simulink model "fuelCycle_Abdou"  (R2022b)
settings: Solver=VariableStepAuto  StartTime=0.0  StopTime=sim_time  RelTol=1e-4
values from neighbouring files (symbols this model uses):
  AF = 90    [BOTH_scenario_inputData.m]    (also in FC_scenario_inputData.m; PO_scenario_inputData.m = 0.7; inputData.m = 70; parametric_analysis_AF.m = AF_array(i))
  eta2 = 0.95    [BOTH_scenario_inputData.m]    (also in FC_scenario_inputData.m; PO_scenario_inputData.m; inputData.m; parametric_analysis_eta_tes.m = eta_tes_array(i))
  f53 = 0.33    [BOTH_scenario_inputData.m]    (also in FC_scenario_inputData.m; PO_scenario_inputData.m; inputData.m; worst_case_InputData.m)
  f54 = 1 - f51 - f53 - f56    (= 0.3399)    [BOTH_scenario_inputData.m]    (also in FC_scenario_inputData.m; PO_scenario_inputData.m; inputData.m; worst_case_InputData.m)
  f56 = 1e-4    (= 0.0001)    [BOTH_scenario_inputData.m]    (also in FC_scenario_inputData.m; PO_scenario_inputData.m; inputData.m; worst_case_InputData.m)
  f96 = 0.1    [BOTH_scenario_inputData.m]    (also in FC_scenario_inputData.m; PO_scenario_inputData.m; inputData.m; worst_case_InputData.m)
  f_dir = 0.7    [BOTH_scenario_inputData.m]    (also in FC_scenario_inputData.m; PO_scenario_inputData.m = 0.3; inputData.m = 0.3; parametric_analysis_f_dir.m = f_dir_array(i))
  fp3 = 1e-4    (= 0.0001)    [BOTH_scenario_inputData.m]    (also in FC_scenario_inputData.m; PO_scenario_inputData.m; inputData.m; parametric_analysis_f_p.m = f_p(i) / 2)
  fp4 = 1e-4    (= 0.0001)    [BOTH_scenario_inputData.m]    (also in FC_scenario_inputData.m; PO_scenario_inputData.m; inputData.m; parametric_analysis_f_p.m = f_p(i) / 2)
  I_s_0 = 1.4    [fuelCycleSimulator.m]    (also in parametric_analysis_AF.m = 0.8; parametric_analysis_epsi.m = 0.8; parametric_analysis_eta_tes.m = 0.8; parametric_analysis_f_dir.m = 0.8)
  lambda = 1.73e-9    (= 1.73e-09)    [BOTH_scenario_inputData.m]    (also in FC_scenario_inputData.m; PO_scenario_inputData.m; inputData.m; worst_case_InputData.m)
  N_dot = 8.99e-7    (= 8.99e-07)    [BOTH_scenario_inputData.m]    (also in FC_scenario_inputData.m = 9.3e-07; PO_scenario_inputData.m = 9.3e-07; inputData.m; worst_case_InputData.m = 9.3e-07)
  T1 = 1/((1 + epsi)/tau1 + lambda)    [BOTH_scenario_inputData.m]    (also in FC_scenario_inputData.m; PO_scenario_inputData.m; inputData.m; parametric_analysis_epsi.m)
  T12 = 1/((1 + epsi)/tau12 + lambda)    [BOTH_scenario_inputData.m]    (also in FC_scenario_inputData.m; PO_scenario_inputData.m; inputData.m; parametric_analysis_epsi.m)
  T2 = 1/((1 + epsi)/tau2 + lambda)    [BOTH_scenario_inputData.m]    (also in FC_scenario_inputData.m; PO_scenario_inputData.m; inputData.m; parametric_analysis_epsi.m)
  T3 = 1/((1 + 0)/tau3 + lambda)    [BOTH_scenario_inputData.m]    (also in FC_scenario_inputData.m; PO_scenario_inputData.m; inputData.m; parametric_analysis_epsi.m)
  T4 = 1/((1 + 0)/tau4 + lambda)    [BOTH_scenario_inputData.m]    (also in FC_scenario_inputData.m; PO_scenario_inputData.m; inputData.m; parametric_analysis_epsi.m)
  T7 = 1/((1 + epsi)/tau7 + lambda)    [BOTH_scenario_inputData.m]    (also in FC_scenario_inputData.m; PO_scenario_inputData.m; inputData.m; parametric_analysis_epsi.m)
  T9 = 1/((1 + epsi)/tau9 + lambda)    [BOTH_scenario_inputData.m]    (also in FC_scenario_inputData.m; PO_scenario_inputData.m; inputData.m; parametric_analysis_TBE.m)
  tau1 = 1.25*3600    (= 4500)    [BOTH_scenario_inputData.m]    (also in FC_scenario_inputData.m; PO_scenario_inputData.m; inputData.m; parametric_analysis_t_blanket.m = tau1_array(i))
  tau12 = 100    [BOTH_scenario_inputData.m]    (also in FC_scenario_inputData.m; PO_scenario_inputData.m; inputData.m; worst_case_InputData.m)
  tau2 = 1*24*3600    (= 86400)    [BOTH_scenario_inputData.m]    (also in FC_scenario_inputData.m; PO_scenario_inputData.m; inputData.m; worst_case_InputData.m)
  tau3 = 1000    [BOTH_scenario_inputData.m]    (also in FC_scenario_inputData.m; PO_scenario_inputData.m; inputData.m; worst_case_InputData.m)
  tau4 = 1000    [BOTH_scenario_inputData.m]    (also in FC_scenario_inputData.m; PO_scenario_inputData.m; inputData.m; worst_case_InputData.m)
  tau5 = 1000    [BOTH_scenario_inputData.m]    (also in FC_scenario_inputData.m; PO_scenario_inputData.m; inputData.m; worst_case_InputData.m)
  tau6 = 3600    [BOTH_scenario_inputData.m]    (also in FC_scenario_inputData.m; PO_scenario_inputData.m; inputData.m; worst_case_InputData.m)
  tau7 = 600    [BOTH_scenario_inputData.m]    (also in FC_scenario_inputData.m; PO_scenario_inputData.m; inputData.m; worst_case_InputData.m)
  tau8 = 0.1*3600    (= 360)    [BOTH_scenario_inputData.m]    (also in FC_scenario_inputData.m; PO_scenario_inputData.m; inputData.m = 3600; parametric_analysis_TBE.m = t_p*0.1)
  tau9 = 0.9*3600    (= 3240)    [BOTH_scenario_inputData.m]    (also in FC_scenario_inputData.m; PO_scenario_inputData.m = 14040; inputData.m = 10800; parametric_analysis_TBE.m = t_p*0.9)
  TBE = 0.1    [BOTH_scenario_inputData.m]    (also in FC_scenario_inputData.m = 0.02; PO_scenario_inputData.m; inputData.m = 0.02; parametric_analysis_AF.m = TBE_array(j))
  TBR = 1.07    [fuelCycleSimulator.m]    (also in parametric_analysis_AF.m = 1; parametric_analysis_TBE.m = 1; parametric_analysis_epsi.m = 1; parametric_analysis_eta_tes.m = 1)
libraries: arc x3
settings Model: SimulationMode=accelerator  Creator=smesc  LastModifiedBy=meschini.samuele
settings SolverCC: InitialStep=1e-4  ShapePreserveControl=EnableAll
settings ModelReferenceCC: EnableRefExpFcnMdlSchedulingChecks=on

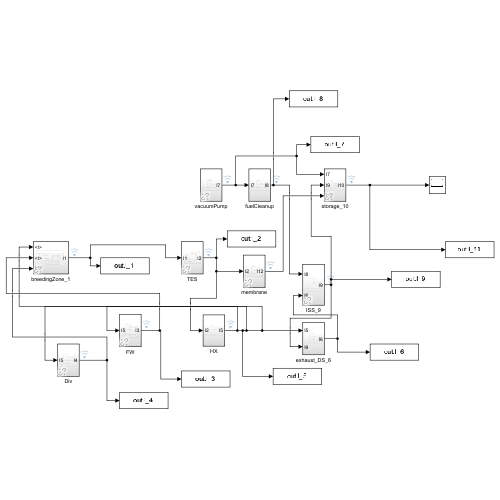
[thumbnail: Simulink's stored preview of the top-level diagram]
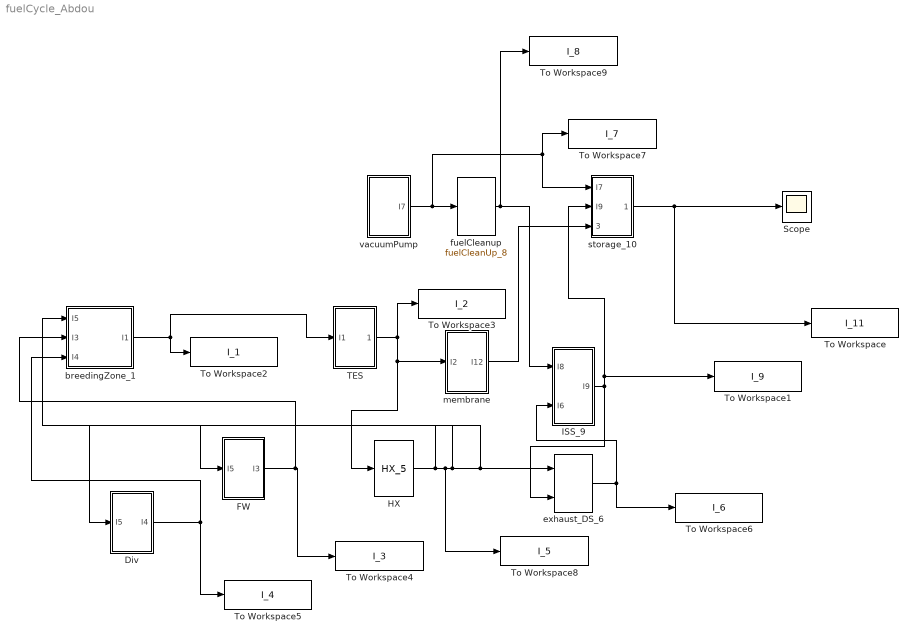
== system fuelCycle_Abdou ==
  Div : Subsystem  AncestorBlock=arc/divertor_4
      settings: LibrarySourceBlock=arc/divertor_4
  FW : Subsystem  AncestorBlock=arc/FW_3
      settings: LibrarySourceBlock=arc/FW_3
  HX : arc/HX_5  SystemSampleTime=-1  VariantActivationTime=update diagram  Latency=0  AutoFrameSizeCalculation=off
      settings: SourceProductName=ARC components
  ISS_9 : Subsystem  AncestorBlock=arc/ISS_9
      settings: LibrarySourceBlock=arc/ISS_9
  Scope : Scope
  TES : Subsystem  AncestorBlock=arc/TES_2
      settings: LibrarySourceBlock=arc/TES_2
  To Workspace : ToWorkspace  VariableName=I_11  SampleTime=-1
  To Workspace1 : ToWorkspace  VariableName=I_9  SampleTime=-1
  To Workspace2 : ToWorkspace  VariableName=I_1  SampleTime=-1
  To Workspace3 : ToWorkspace  VariableName=I_2  SampleTime=-1
  To Workspace4 : ToWorkspace  VariableName=I_3  SampleTime=-1
  To Workspace5 : ToWorkspace  VariableName=I_4  SampleTime=-1
  To Workspace6 : ToWorkspace  VariableName=I_6  SampleTime=-1
  To Workspace7 : ToWorkspace  VariableName=I_7  SampleTime=-1
  To Workspace8 : ToWorkspace  VariableName=I_5  SampleTime=-1
  To Workspace9 : ToWorkspace  VariableName=I_8  SampleTime=-1
  breedingZone_1 : Subsystem  AncestorBlock=arc/breedingZone_1
      settings: LibrarySourceBlock=arc/breedingZone_1
  exhaust_DS_6 : arc/exhaust_DS_6  SystemSampleTime=-1  VariantActivationTime=update diagram  Latency=0  AutoFrameSizeCalculation=off
      link override Gain: Gain=f56/tau5
      settings: SourceProductName=ARC components
  fuelCleanup : arc/fuelCleanUp_8  SystemSampleTime=-1  VariantActivationTime=update diagram  Latency=0  AutoFrameSizeCalculation=off
      settings: SourceProductName=ARC components
  membrane : Subsystem  AncestorBlock=arc/fuelCleanUp_8
      settings: LibrarySourceBlock=arc/fuelCleanUp_8
  storage_10 : Subsystem  AncestorBlock=arc/storage_10
      settings: LibrarySourceBlock=arc/storage_10
  vacuumPump : Subsystem  AncestorBlock=arc/pump_7
      settings: LibrarySourceBlock=arc/pump_7
  wires:
  breedingZone_1/1(I1) -> TES/1(I1), To Workspace2/1
  TES/1(Output) -> To Workspace3/1, membrane/1(I2), HX/1
  HX/1 -> FW/1(I5), To Workspace8/1, Div/1(I5), exhaust_DS_6/1, breedingZone_1/1(I5)
  exhaust_DS_6/1 -> ISS_9/2(I6), To Workspace6/1
  ISS_9/1(I9) -> exhaust_DS_6/2, storage_10/2(I9), To Workspace1/1
  vacuumPump/1(I7) -> To Workspace7/1, storage_10/1(I7), fuelCleanup/1
  fuelCleanup/1 -> To Workspace9/1, ISS_9/1(I8)
  storage_10/1(I10) -> To Workspace/1, Scope/1
  FW/1(I3) -> breedingZone_1/2(I3), To Workspace4/1
  Div/1(I4) -> breedingZone_1/3(I4), To Workspace5/1
  membrane/1(I12) -> storage_10/3(I12)

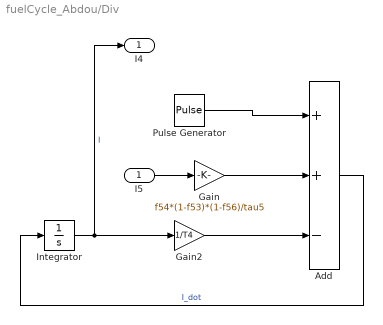
== system fuelCycle_Abdou/Div ==
  I5 : Inport
  Add : Sum  Inputs=++-
  Gain : Gain  Gain=f54*(1-f53)*(1-f56)/tau5
  Gain2 : Gain  Gain=1/T4
  Integrator : Integrator
  Pulse Generator : DiscretePulseGenerator  PulseType=Time based  Amplitude=fp4*N_dot/TBE  Period=1800  PulseWidth=AF
  I4 : Outport
  wires:
  Pulse Generator/1 -> Add/1
  Gain/1 -> Add/2
  Integrator/1 -> Gain2/1, I4/1  "I"
  Add/1 -> Integrator/1  "I_dot"
  Gain2/1 -> Add/3
  I5/1 -> Gain/1

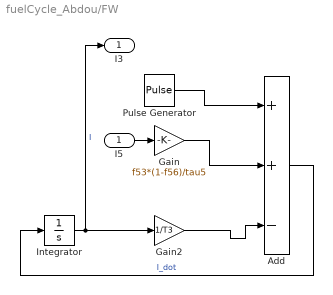
== system fuelCycle_Abdou/FW ==
  I5 : Inport
  Add : Sum  Inputs=++-
  Gain : Gain  Gain=f53*(1-f56)/tau5
  Gain2 : Gain  Gain=1/T3
  Integrator : Integrator
  Pulse Generator : DiscretePulseGenerator  PulseType=Time based  Amplitude=fp3*N_dot/TBE  Period=1800  PulseWidth=AF
  I3 : Outport
  wires:
  Gain2/1 -> Add/3
  Pulse Generator/1 -> Add/1
  Integrator/1 -> I3/1, Gain2/1  "I"
  Add/1 -> Integrator/1  "I_dot"
  Gain/1 -> Add/2
  I5/1 -> Gain/1

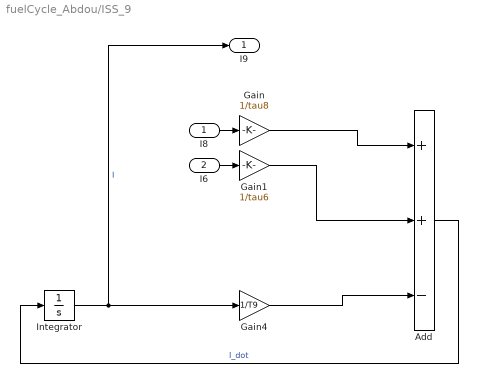
== system fuelCycle_Abdou/ISS_9 ==
  I8 : Inport
  I6 : Inport  Port=2
  Add : Sum  Inputs=++-
  Gain : Gain  Gain=1/tau8
  Gain1 : Gain  Gain=1/tau6
  Gain4 : Gain  Gain=1/T9
  Integrator : Integrator
  I9 : Outport
  wires:
  I8/1 -> Gain/1
  Gain1/1 -> Add/2
  I6/1 -> Gain1/1
  Add/1 -> Integrator/1  "I_dot"
  Integrator/1 -> Gain4/1, I9/1  "I"
  Gain/1 -> Add/1
  Gain4/1 -> Add/3

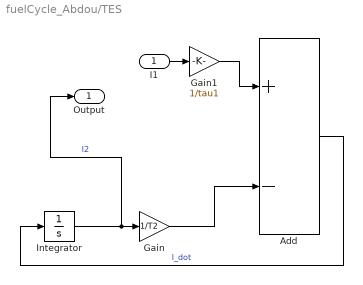
== system fuelCycle_Abdou/TES ==
  I1 : Inport
  Add : Sum  Inputs=+-
  Gain : Gain  Gain=1/T2
  Gain1 : Gain  Gain=1/tau1
  Integrator : Integrator
  Output : Outport
  wires:
  Gain/1 -> Add/2
  I1/1 -> Gain1/1
  Gain1/1 -> Add/1
  Integrator/1 -> Gain/1, Output/1  "I2"
  Add/1 -> Integrator/1  "I_dot"

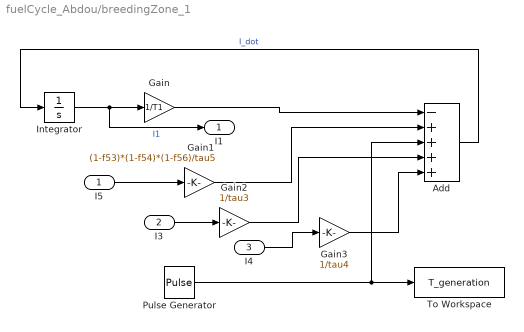
== system fuelCycle_Abdou/breedingZone_1 ==
  I5 : Inport
  I3 : Inport  Port=2
  I4 : Inport  Port=3
  Add : Sum  Inputs=-++++
  Gain : Gain  Gain=1/T1
  Gain1 : Gain  Gain=(1-f53)*(1-f54)*(1-f56)/tau5
  Gain2 : Gain  Gain=1/tau3
  Gain3 : Gain  Gain=1/tau4
  Integrator : Integrator
  Pulse Generator : DiscretePulseGenerator  PulseType=Time based  Amplitude=N_dot * TBR  Period=1800  PulseWidth=AF
  To Workspace : ToWorkspace  VariableName=T_generation  SaveFormat=Timeseries  SampleTime=-1
  I1 : Outport
  wires:
  Add/1 -> Integrator/1  "I_dot"
  Gain1/1 -> Add/2
  Integrator/1 -> Gain/1, I1/1  "I1"
  Gain/1 -> Add/1
  I5/1 -> Gain1/1
  Pulse Generator/1 -> Add/3, To Workspace/1
  I3/1 -> Gain2/1
  Gain2/1 -> Add/4
  I4/1 -> Gain3/1
  Gain3/1 -> Add/5

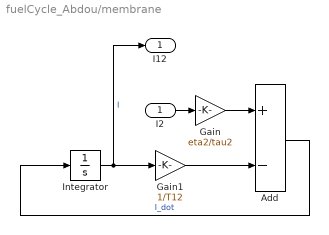
== system fuelCycle_Abdou/membrane ==
  I2 : Inport
  Add : Sum  Inputs=+-
  Gain : Gain  Gain=eta2/tau2
  Gain1 : Gain  Gain=1/T12
  Integrator : Integrator
  I12 : Outport
  wires:
  I2/1 -> Gain/1
  Gain1/1 -> Add/2
  Add/1 -> Integrator/1  "I_dot"
  Integrator/1 -> Gain1/1, I12/1  "I"
  Gain/1 -> Add/1

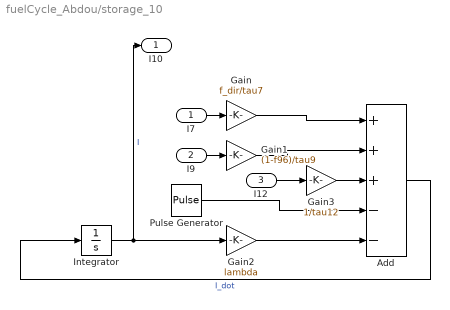
== system fuelCycle_Abdou/storage_10 ==
  I7 : Inport
  I9 : Inport  Port=2
  I12 : Inport  Port=3
  Add : Sum  Inputs=+++--
  Gain : Gain  Gain=f_dir/tau7
  Gain1 : Gain  Gain=(1-f96)/tau9
  Gain2 : Gain  Gain=lambda
  Gain3 : Gain  Gain=1/tau12
  Integrator : Integrator  InitialCondition=I_s_0
  Pulse Generator : DiscretePulseGenerator  PulseType=Time based  Amplitude=N_dot/TBE  Period=1800  PulseWidth=AF
  I10 : Outport
  wires:
  Integrator/1 -> Gain2/1, I10/1  "I"
  I9/1 -> Gain1/1
  Add/1 -> Integrator/1  "I_dot"
  Gain2/1 -> Add/5
  I7/1 -> Gain/1
  Gain1/1 -> Add/2
  Gain/1 -> Add/1
  Pulse Generator/1 -> Add/4
  I12/1 -> Gain3/1
  Gain3/1 -> Add/3

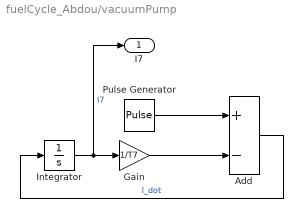
== system fuelCycle_Abdou/vacuumPump ==
  Add : Sum  Inputs=+-
  Gain : Gain  Gain=1/T7
  Integrator : Integrator
  Pulse Generator : DiscretePulseGenerator  PulseType=Time based  Amplitude=(1-TBE-fp3-fp4)*N_dot/TBE  Period=1800  PulseWidth=AF
  I7 : Outport
  wires:
  Gain/1 -> Add/2
  Integrator/1 -> Gain/1, I7/1  "I7"
  Pulse Generator/1 -> Add/1
  Add/1 -> Integrator/1  "I_dot"
